simulink model "ros_test"  (R2025b)
settings: Solver=VariableStepAuto  StartTime=0.0  StopTime=inf  RelTol=1e-3
libraries: ros2lib x3
settings Model: Creator=vulcangrip  LastModifiedBy=vulcangrip

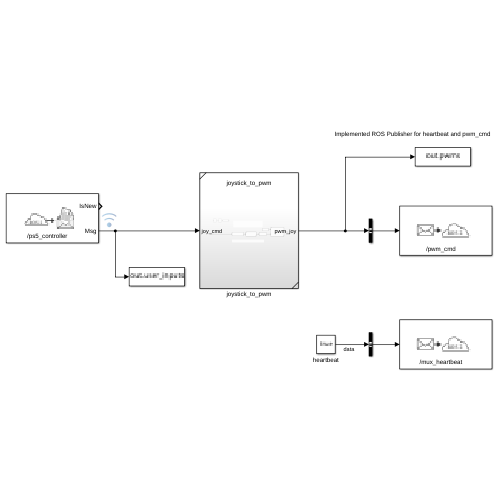
[thumbnail: Simulink's stored preview of the top-level diagram]
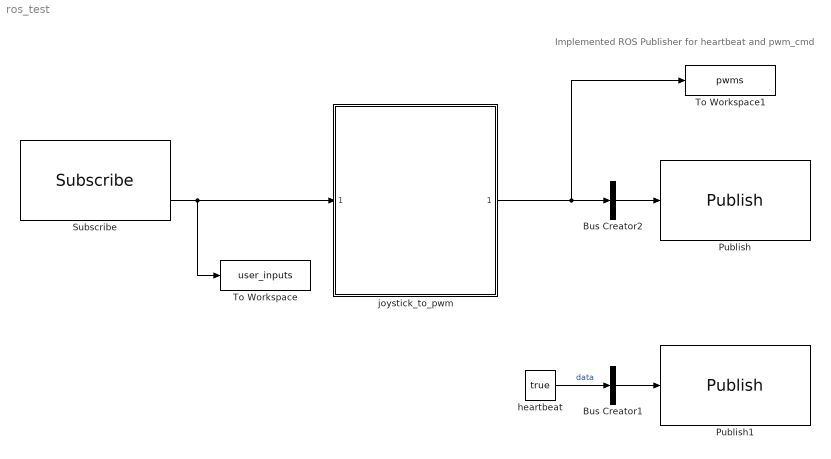
== system ros_test ==
  note: Implemented ROS Publisher for heartbeat and pwm_cmd
  Bus Creator1 : BusCreator  Inputs=1
  Bus Creator2 : BusCreator  Inputs=1
  Publish : ros2lib/Publish  topicSource=Specify your own  topic=/pwm_cmd  messageType=custom_interfaces/Pwms  QOSHistory=Keep last  QOSDepth=10  QOSReliability=Reliable  QOSDurability=Volatile  QOSDeadline=Inf  QOSLifespan=Inf  QOSLiveliness=Automatic  QOSLeaseDuration=Inf  QOSAvoidROSNamespaceConventions=off
  Publish1 : ros2lib/Publish  topicSource=Specify your own  topic=/mux_heartbeat  messageType=std_msgs/Bool  QOSHistory=Keep last  QOSDepth=10  QOSReliability=Reliable  QOSDurability=Volatile  QOSDeadline=Inf  QOSLifespan=Inf  QOSLiveliness=Automatic  QOSLeaseDuration=Inf  QOSAvoidROSNamespaceConventions=off
  Subscribe : ros2lib/Subscribe  topicSource=Specify your own  topic=/ps5_controller  messageType=remote_control_interface/Gamepad  sampleTime=1/60  QOSHistory=Keep last  QOSDepth=10  QOSReliability=Reliable  QOSDurability=Volatile  QOSDeadline=Inf  QOSLifespan=Inf  QOSLiveliness=Automatic  QOSLeaseDuration=Inf  QOSAvoidROSNamespaceConventions=off
  To Workspace : ToWorkspace  VariableName=user_inputs  SaveFormat=Timeseries  SampleTime=-1
  To Workspace1 : ToWorkspace  VariableName=pwms  SaveFormat=Timeseries  SampleTime=-1
  heartbeat : Constant  Value=true
  joystick_to_pwm : Subsystem  ReferencedSubsystem=joystick_to_pwm
  wires:
  Subscribe/2 -> To Workspace/1, joystick_to_pwm/1
  joystick_to_pwm/1 -> To Workspace1/1, Bus Creator2/1
  heartbeat/1 -> Bus Creator1/1  "data"
  Bus Creator1/1 -> Publish1/1
  Bus Creator2/1 -> Publish/1
